simulink model "ejemploDB"  (R2018a)
settings: Solver=VariableStepAuto  StartTime=0.0  StopTime=10.0  RelTol=1e-3
values from neighbouring files (symbols this model uses):
  A = [0 1 0 0 ... (first row only)    [ejemplo_ft.m]    (also in ft.m = [0 1; -5/3 0])
  B = [0 0 0 1]'    [ejemplo_ft.m]    (also in ft.m = [0 5/3]')
  C = [1 0 0 0]    [ejemplo_ft.m]    (also in ft.m = [1 0])
settings Model: Creator=carma  LastModifiedBy=carma

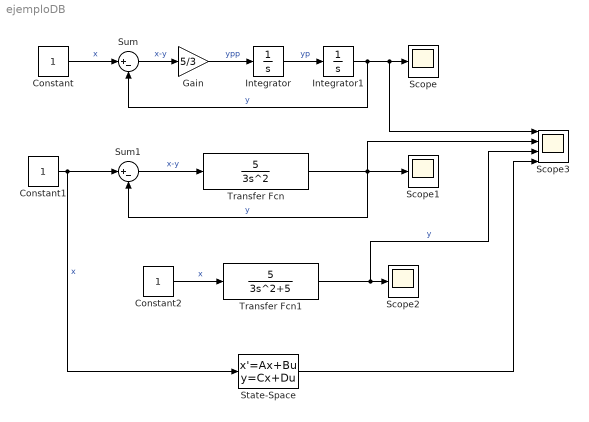
== system ejemploDB ==
  Constant : Constant
  Constant1 : Constant
  Constant2 : Constant
  Gain : Gain  Gain=5/3
  Integrator : Integrator
  Integrator1 : Integrator
  Scope : Scope
  Scope1 : Scope
  Scope2 : Scope
  Scope3 : Scope  NumInputPorts=4
  State-Space : StateSpace  A=A  B=B  C=C  D=0  InitialCondition=0
  Sum : Sum  Inputs=|+-
  Sum1 : Sum  Inputs=|+-
  Transfer Fcn : TransferFcn  Numerator=[5]  Denominator=[3 0 0]
  Transfer Fcn1 : TransferFcn  Numerator=[5]  Denominator=[3 0 5]
  wires:
  Sum/1 -> Gain/1  "x-y"
  Constant/1 -> Sum/1  "x"
  Integrator1/1 -> Scope3/1, Scope/1, Sum/2  "y"
  Gain/1 -> Integrator/1  "ypp"
  Integrator/1 -> Integrator1/1  "yp"
  Transfer Fcn/1 -> Scope3/2, Scope1/1, Sum1/2  "y"
  Sum1/1 -> Transfer Fcn/1  "x-y"
  Constant1/1 -> State-Space/1, Sum1/1  "x"
  Constant2/1 -> Transfer Fcn1/1  "x"
  Transfer Fcn1/1 -> Scope3/3, Scope2/1  "y"
  State-Space/1 -> Scope3/4
